simulink model "TV_2017"  (R2016a)
settings: Solver=FixedStepAuto  StartTime=0.0  StopTime=inf  FixedStep=0.001  RelTol=1e-3
PreLoadFcn:
  | TV_2017_parameters
values from neighbouring files (symbols this model uses):
  battery_voltage = single(530)    [HIL_parameters.m]    (also in HIL_parameters_2018.m; TV_2017_parameters.m; TV_2017_parameters_VD.m)
  car_params = Simulink_Car_params    [HIL_parameters.m]    (also in HIL_parameters_2018.m; TV_2017_parameters.m; TV_2017_parameters_VD.m)
  i_Diff = 16    [HIL_parameters.m]    (also in HIL_parameters_2018.m; TV_2017_parameters.m)
  Kp = 1    [HIL_parameters.m]    (also in HIL_parameters_2018.m; TV_2017_parameters.m; TV_2017_parameters_VD.m)
  motor_data = struct    [HIL_parameters.m]    (also in HIL_parameters_2018.m; TV_2017_parameters.m)
  powerLimitControl = Simulink_el    [HIL_parameters.m]    (also in HIL_parameters_2018.m; TV_2017_parameters.m; TV_2017_parameters_VD.m)
  settings = Simulink_Settings    [HIL_parameters.m]    (also in HIL_parameters_2018.m; TV_2017_parameters.m; TV_2017_parameters_VD.m)
  SpdC_BCC = 0    [HIL_parameters.m]    (also in HIL_parameters_2018.m; TV_2017_parameters.m; TV_2017_parameters_VD.m)
  Speed_Neg_sat = -21    [HIL_parameters.m]    (also in HIL_parameters_2018.m; TV_2017_parameters.m; TV_2017_parameters_VD.m)
  Speed_Pos_sat = 21    [HIL_parameters.m]    (also in HIL_parameters_2018.m; TV_2017_parameters.m; TV_2017_parameters_VD.m)
  SteeringAngleFL = [-23.80 -22.65 -21.50 -20.34 -19.18 -18.03 -16.86 -15.70 -14.53 -13.35 -12.18 -10.99 -9.80 -8.61 -7.40 -6.19 -4.97 -3.75 -2.51 -1.26 0 1.27 2.56 3.85 5.17 6.50 7.84 9.21 10.59 12.00 13.42 14.88 16.36 17.87 19.41 20.99 22.61 24.26 25.97 27.73 29.54]    [CarSetupAnalysis2018.m]    (also in HIL_parameters_2018.m; TV_2017_parameters.m; TV_2017_parameters_VD.m = [-24.129 -22.950 -21.772 -20.593 -19.413 -18.232 -17.050 -15)
  SteeringAngleFR = [-29.54 -27.73 -25.97 -24.26 -22.61 -20.99 -19.41 -17.87 -16.36 -14.88 -13.42 -12.00 -10.59 -9.21 -7.84 -6.50 -5.17 -3.85 -2.56 -1.27 0 1.26 2.51 3.75 4.97 6.19 7.40 8.61 9.80 10.99 12.18 13.35 14.53 15.70 16.86 18.03 19.18 20.34 21.50 22.65 23.80]    [CarSetupAnalysis2018.m]    (also in HIL_parameters_2018.m; TV_2017_parameters.m; TV_2017_parameters_VD.m = [-29.3050 -27.5340 -25.8140 -24.1410 -22.5110 -20.9180 -19.3)
  SteeringWhAngle = [-105 -99.75 -94.5 -89.25 -84 -78.75 -73.5 -68.25 -63 -57.75 -52.5 -47.25 -42 -36.75 -31.5 -26.25 -21.0 -15.75 -10.5 -5.25 0.0 5.25 10.50 15.75 21.00 26.25 31.50 36.75 42.00 47.25 52.50 57.75  63.00 68.25 73.50 78.75 84.00 89.25 94.50 99.75 105.00]    [TV_2017_parameters_VD.m]
  Tn_n = 0    [HIL_parameters.m]    (also in HIL_parameters_2018.m; TV_2017_parameters.m; TV_2017_parameters_VD.m)
  tractionControl = Simulink_tc    [HIL_parameters.m]    (also in HIL_parameters_2018.m; IterativeTractionControlTuning.m; TV_2017_parameters.m; TV_2017_parameters_VD.m)
  yawMomentGenerator = struct    [HIL_parameters.m]    (also in HIL_parameters_2018.m = Simulink_yawRate2; TV_2017_parameters.m = Simulink_yawRate2)
  yawRateControl = Simulink_yawRate    [HIL_parameters.m]    (also in HIL_parameters_2018.m; TV_2017_parameters.m; TV_2017_parameters_VD.m)
undefined symbols (not defined in the file or in its folder): DiscIntNeverNeededParam, magnitude, speedEstimation, TC_Decr_Gas, TC_Derivative, TC_Incr_Gas, TC_On, TC_Relay_Off, TC_Relay_On
libraries: CarMaker4SL x350, simulink_extras x63, simulink x37, dspfdesign x2
(part 3 of 14)

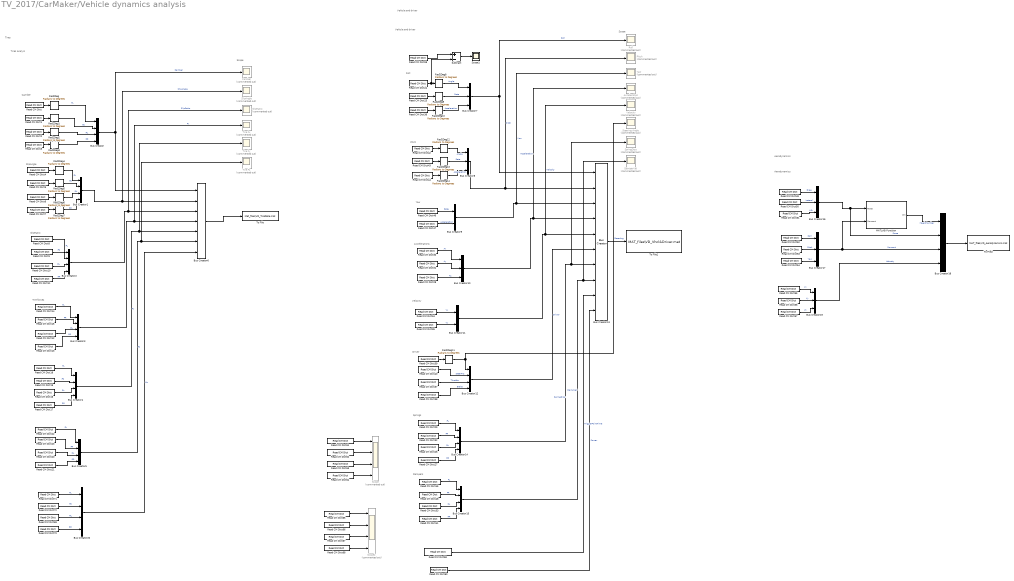
== system TV_2017/CarMaker/Vehicle dynamics analysis ==
  note: Aerodynamics
  note: Scope
  note: Scope
  note: Dampers
  note: Springs
  note: Driver
  note: Velocity
  note: Tire forces
  note: SlipRatio
  note: SlipAngle
  note: Camber
  note: Tires analyis
  note: Tires
  note: Accelerations
  note: Yaw
  note: Pitch
  note: Roll
  note: Vehicle and driver
  note: Vehicle and driver
  note: Aerodynamics
  Acceleration : Scope  Commented=on
  Bus Creator{,1..5,12,14..15,18,20} (11 alike) : BusCreator  Inputs=4
  Bus Creator{7..8,10,16..17,19} (6 alike) : BusCreator  Inputs=3
  Bus Creator11 : BusCreator  Inputs=2
  Bus Creator13 : BusCreator  Inputs=10
  Bus Creator6 : BusCreator  Inputs=7
  Bus Creator9 : BusCreator  Inputs=2
  Camber : Scope  Commented=on
  DamperVel : Scope  Commented=on
  MATLAB Function : MATLAB Function  TreatAsAtomicUnit=on
  Pitch : Scope  Commented=on
  Rad2Deg{,1..14} (15 alike) : simulink_extras/Transformations/Radians to Degrees
  Read CM Dict : CarMaker4SL/Read CM Dict  xname=Car.CamberFL  xsync=off
  Read CM Dict1 : CarMaker4SL/Read CM Dict  xname=Car.CamberFR  xsync=off
  Read CM Dict10 : CarMaker4SL/Read CM Dict  xname=Vhcl.RL.LongSlip  xsync=off
  Read CM Dict11 : CarMaker4SL/Read CM Dict  xname=Vhcl.RR.LongSlip  xsync=off
  Read CM Dict12 : CarMaker4SL/Read CM Dict  xname=Vhcl.RL.Fx  xsync=off
  Read CM Dict13 : CarMaker4SL/Read CM Dict  xname=Vhcl.RR.Fx  xsync=off
  Read CM Dict14 : CarMaker4SL/Read CM Dict  xname=Vhcl.FL.Fx  xsync=off
  Read CM Dict15 : CarMaker4SL/Read CM Dict  xname=Vhcl.FR.Fx  xsync=off
  Read CM Dict16 : CarMaker4SL/Read CM Dict  xname=Vhcl.RL.Fy  xsync=off
  Read CM Dict17 : CarMaker4SL/Read CM Dict  xname=Vhcl.RR.Fy  xsync=off
  Read CM Dict18 : CarMaker4SL/Read CM Dict  xname=Vhcl.FL.Fy  xsync=off
  Read CM Dict19 : CarMaker4SL/Read CM Dict  xname=Vhcl.FR.Fy  xsync=off
  Read CM Dict2 : CarMaker4SL/Read CM Dict  xname=Car.CamberRL  xsync=off
  Read CM Dict20 : CarMaker4SL/Read CM Dict  xname=Vhcl.RL.Fz  xsync=off
  Read CM Dict21 : CarMaker4SL/Read CM Dict  xname=Vhcl.RR.Fz  xsync=off
  Read CM Dict22 : CarMaker4SL/Read CM Dict  xname=Vhcl.FL.Fz  xsync=off
  Read CM Dict23 : CarMaker4SL/Read CM Dict  xname=Vhcl.FR.Fz  xsync=off
  Read CM Dict24 : CarMaker4SL/Read CM Dict  xname=Vhcl.Roll  xsync=off
  Read CM Dict25 : CarMaker4SL/Read CM Dict  xname=Vhcl.RollVel  xsync=off
  Read CM Dict26 : CarMaker4SL/Read CM Dict  xname=Car.SpringRL.l  xsync=off
  Read CM Dict27 : CarMaker4SL/Read CM Dict  xname=Car.SpringRR.l  xsync=off
  Read CM Dict28 : CarMaker4SL/Read CM Dict  xname=Car.az  xsync=off
  Read CM Dict29 : CarMaker4SL/Read CM Dict  xname=Car.SpringFL.l  xsync=off
  Read CM Dict3 : CarMaker4SL/Read CM Dict  xname=Car.CamberRR  xsync=off
  Read CM Dict30 : CarMaker4SL/Read CM Dict  xname=Car.ax  xsync=off
  Read CM Dict31 : CarMaker4SL/Read CM Dict  xname=Car.ay  xsync=off
  Read CM Dict32 : CarMaker4SL/Read CM Dict  xname=Car.SpringFR.l  xsync=off
  Read CM Dict33 : CarMaker4SL/Read CM Dict  xname=Car.DampRL.v  xsync=off
  Read CM Dict34 : CarMaker4SL/Read CM Dict  xname=Car.vx  xsync=off
  Read CM Dict35 : CarMaker4SL/Read CM Dict  xname=Car.vy  xsync=off
  Read CM Dict36 : CarMaker4SL/Read CM Dict  xname=Vhcl.RollAcc  xsync=off
  Read CM Dict37 : CarMaker4SL/Read CM Dict  xname=Driver.Gas  xsync=off
  Read CM Dict38 : CarMaker4SL/Read CM Dict  xname=Driver.Brake  xsync=off
  Read CM Dict39 : CarMaker4SL/Read CM Dict  xname=Vhcl.Steer.Ang  xsync=off
  Read CM Dict4 : CarMaker4SL/Read CM Dict  xname=Vhcl.FL.SideSlip  xsync=off
  Read CM Dict40 : CarMaker4SL/Read CM Dict  xname=Vhcl.Steer.Trq  xsync=off
  Read CM Dict41 : CarMaker4SL/Read CM Dict  xname=Car.DampRR.v  xsync=off
  Read CM Dict42 : CarMaker4SL/Read CM Dict  xname=Vhcl.Pitch  xsync=off
  Read CM Dict43 : CarMaker4SL/Read CM Dict  xname=Vhcl.PitchVel  xsync=off
  Read CM Dict44 : CarMaker4SL/Read CM Dict  xname=Vhcl.PitchAcc  xsync=off
  Read CM Dict45 : CarMaker4SL/Read CM Dict  xname=Car.DampFL.v  xsync=off
  Read CM Dict46 : CarMaker4SL/Read CM Dict  xname=Vhcl.YawRate  xsync=off
  Read CM Dict47 : CarMaker4SL/Read CM Dict  xname=Vhcl.YawAcc  xsync=off
  Read CM Dict48 : CarMaker4SL/Read CM Dict  xname=Car.DampFR.v  xsync=off
  Read CM Dict49 : CarMaker4SL/Read CM Dict  xname=Car.Aero.Frc_1.x  xsync=off
  Read CM Dict5 : CarMaker4SL/Read CM Dict  xname=Vhcl.FR.SideSlip  xsync=off
  Read CM Dict50 : CarMaker4SL/Read CM Dict  xname=Car.Aero.Frc_1.y  xsync=off
  Read CM Dict51 : CarMaker4SL/Read CM Dict  xname=Car.Aero.Frc_1.z  xsync=off
  Read CM Dict52 : CarMaker4SL/Read CM Dict  xname=Car.Aero.Trq_1.x  xsync=off
  Read CM Dict53 : CarMaker4SL/Read CM Dict  xname=Car.Aero.Trq_1.y  xsync=off
  Read CM Dict54 : CarMaker4SL/Read CM Dict  xname=Car.Aero.Trq_1.z  xsync=off
  Read CM Dict55 : CarMaker4SL/Read CM Dict  xname=Car.Aero.vres_1.x  xsync=off
  Read CM Dict56 : CarMaker4SL/Read CM Dict  xname=Car.Aero.vres_1.y  xsync=off
  Read CM Dict57 : CarMaker4SL/Read CM Dict  xname=Car.Aero.vres_1.z  xsync=off
  Read CM Dict58 : CarMaker4SL/Read CM Dict  xname=DM.TriggerPoint.Time  xsync=off
  Read CM Dict59 : CarMaker4SL/Read CM Dict  xname=Car.Roll  xsync=off
  Read CM Dict6 : CarMaker4SL/Read CM Dict  xname=Vhcl.RL.SideSlip  xsync=off
  Read CM Dict60 : CarMaker4SL/Read CM Dict  xname=Power  xsync=off
  Read CM Dict61 : CarMaker4SL/Read CM Dict  xname=Car.SpringFL.Frc_tot  xsync=off
  Read CM Dict62 : CarMaker4SL/Read CM Dict  xname=Car.SpringFR.Frc_tot  xsync=off
  Read CM Dict63 : CarMaker4SL/Read CM Dict  xname=Car.SpringRL.Frc_tot  xsync=off
  Read CM Dict64 : CarMaker4SL/Read CM Dict  xname=Car.SpringRR.Frc_tot  xsync=off
  Read CM Dict65 : CarMaker4SL/Read CM Dict  xname=Car.DampFL.Frc_tot  xsync=off
  Read CM Dict66 : CarMaker4SL/Read CM Dict  xname=Car.DampFR.Frc_tot  xsync=off
  Read CM Dict67 : CarMaker4SL/Read CM Dict  xname=Car.DampRL.Frc_tot  xsync=off
  Read CM Dict68 : CarMaker4SL/Read CM Dict  xname=Car.DampRR.Frc_tot  xsync=off
  Read CM Dict69 : CarMaker4SL/Read CM Dict  xname=Car.TrqAlignRL  xsync=off
  Read CM Dict7 : CarMaker4SL/Read CM Dict  xname=Vhcl.RR.SideSlip  xsync=off
  Read CM Dict70 : CarMaker4SL/Read CM Dict  xname=Car.TrqAlignRR  xsync=off
  Read CM Dict71 : CarMaker4SL/Read CM Dict  xname=Car.TrqAlignFL  xsync=off
  Read CM Dict72 : CarMaker4SL/Read CM Dict  xname=Car.TrqAlignFR  xsync=off
  Read CM Dict8 : CarMaker4SL/Read CM Dict  xname=Vhcl.FL.LongSlip  xsync=off
  Read CM Dict9 : CarMaker4SL/Read CM Dict  xname=Vhcl.FR.LongSlip  xsync=off
  Roll : Scope  Commented=on
  Scope : Scope  Commented=on  NumInputPorts=4
  Scope1 : Scope
  Scope2 : Scope  Commented=on  NumInputPorts=4
  SlipAngle : Scope  Commented=on
  SlipRatio : Scope  Commented=on
  SpringDisp : Scope  Commented=on
  Steering Angle : Scope  Commented=on
  Subtract : Sum  Inputs=+-
  Tire Fx : Scope  Commented=on
  Tire Fy : Scope  Commented=on
  Tire Fz : Scope  Commented=on
  To File : ToFile  Filename=Mat_files\VD_TireData.mat  MatrixName=Tire  SaveFormat=Timeseries
      settings: Decimation=2
  To File1 : ToFile  Filename=MAT_files\VD_Vhcl&Driver.mat  MatrixName=Vhcl  SaveFormat=Timeseries
      settings: Decimation=2
  To File2 : ToFile  Filename=MAT_files\VD_Aerodynamics.mat  MatrixName=Aero  SaveFormat=Timeseries
      settings: Decimation=2
  Velocity : Scope  Commented=on
  Yaw : Scope  Commented=on
  wires:
  Rad2Deg3/1 -> Bus Creator/4  "RR"
  Read CM Dict2/1 -> Rad2Deg2/1
  Rad2Deg/1 -> Bus Creator/1  "FL"
  Rad2Deg2/1 -> Bus Creator/3  "RL"
  Read CM Dict/1 -> Rad2Deg/1
  Rad2Deg1/1 -> Bus Creator/2  "FR"
  Read CM Dict1/1 -> Rad2Deg1/1
  Read CM Dict3/1 -> Rad2Deg3/1
  Rad2Deg7/1 -> Bus Creator1/4  "RR"
  Read CM Dict6/1 -> Rad2Deg6/1
  Rad2Deg4/1 -> Bus Creator1/1  "FL"
  Rad2Deg6/1 -> Bus Creator1/3  "RL"
  Read CM Dict4/1 -> Rad2Deg4/1
  Rad2Deg5/1 -> Bus Creator1/2  "FR"
  Read CM Dict5/1 -> Rad2Deg5/1
  Read CM Dict7/1 -> Rad2Deg7/1
  Read CM Dict11/1 -> Bus Creator2/4  "RR"
  Read CM Dict8/1 -> Bus Creator2/1  "FL"
  Read CM Dict10/1 -> Bus Creator2/3  "RL"
  Read CM Dict9/1 -> Bus Creator2/2  "FR"
  Read CM Dict13/1 -> Bus Creator3/4  "RR"
  Read CM Dict14/1 -> Bus Creator3/1  "FL"
  Read CM Dict12/1 -> Bus Creator3/3  "RL"
  Read CM Dict15/1 -> Bus Creator3/2  "FR"
  Read CM Dict17/1 -> Bus Creator4/4  "RR"
  Read CM Dict18/1 -> Bus Creator4/1  "FL"
  Read CM Dict16/1 -> Bus Creator4/3  "RL"
  Read CM Dict19/1 -> Bus Creator4/2  "FR"
  Read CM Dict21/1 -> Bus Creator5/4  "RR"
  Read CM Dict22/1 -> Bus Creator5/1  "FL"
  Read CM Dict20/1 -> Bus Creator5/3  "RL"
  Bus Creator/1 -> Bus Creator6/1, Camber/1  "Camber"
  Bus Creator1/1 -> SlipAngle/1, Bus Creator6/2  "SlipAngle"
  Bus Creator2/1 -> SlipRatio/1, Bus Creator6/3  "SlipRatio"
  Bus Creator3/1 -> Bus Creator6/4, Tire Fx/1  "Fx"
  Bus Creator4/1 -> Tire Fy/1, Bus Creator6/5  "Fy"
  Bus Creator5/1 -> Tire Fz/1, Bus Creator6/6  "Fz"
  Read CM Dict23/1 -> Bus Creator5/2  "FR"
  Bus Creator6/1 -> To File/1
  Read CM Dict36/1 -> Rad2Deg10/1
  Rad2Deg8/1 -> Bus Creator7/1  "Angle"
  Rad2Deg10/1 -> Bus Creator7/3  "Acceleration"
  Read CM Dict24/1 -> Subtract/2, Rad2Deg8/1
  Rad2Deg9/1 -> Bus Creator7/2  "Rate"
  Read CM Dict25/1 -> Rad2Deg9/1
  Read CM Dict44/1 -> Rad2Deg14/1
  Rad2Deg12/1 -> Bus Creator8/1  "Angle"
  Rad2Deg14/1 -> Bus Creator8/3  "Acceleration"
  Read CM Dict42/1 -> Rad2Deg12/1
  Rad2Deg13/1 -> Bus Creator8/2  "Rate"
  Read CM Dict43/1 -> Rad2Deg13/1
  Read CM Dict46/1 -> Bus Creator9/1  "Rate"
  Read CM Dict47/1 -> Bus Creator9/2  "Acceleration"
  Read CM Dict34/1 -> Bus Creator11/1  "Vx"
  Read CM Dict35/1 -> Bus Creator11/2  "Vy"
  Read CM Dict38/1 -> Bus Creator12/4  "Brake"
  Read CM Dict39/1 -> Rad2Deg11/1
  Read CM Dict37/1 -> Bus Creator12/3  "Throttle"
  Bus Creator7/1 -> Bus Creator13/1, Roll/1  "Roll"
  Bus Creator8/1 -> Pitch/1, Bus Creator13/2  "Pitch"
  Bus Creator9/1 -> Bus Creator13/3, Yaw/1  "Yaw"
  Bus Creator11/1 -> Velocity/1, Bus Creator13/5  "Velocity"
  Bus Creator12/1 -> Bus Creator13/6  "Driver"
  Read CM Dict40/1 -> Bus Creator12/2  "SteerTrq"
  Bus Creator13/1 -> To File1/1
  Rad2Deg11/1 -> Bus Creator12/1, Steering Angle/1  "SteerAng"
  Bus Creator10/1 -> Acceleration/1, Bus Creator13/4  "Acceleration"
  Read CM Dict27/1 -> Bus Creator14/4  "RR"
  Read CM Dict29/1 -> Bus Creator14/1  "FL"
  Read CM Dict26/1 -> Bus Creator14/3  "RL"
  Read CM Dict32/1 -> Bus Creator14/2  "FR"
  Bus Creator14/1 -> SpringDisp/1, Bus Creator13/7  "SpringDisp"
  Read CM Dict41/1 -> Bus Creator15/4  "RR"
  Read CM Dict45/1 -> Bus Creator15/1  "FL"
  Read CM Dict33/1 -> Bus Creator15/3  "RL"
  Read CM Dict48/1 -> Bus Creator15/2  "FR"
  Bus Creator15/1 -> DamperVel/1, Bus Creator13/8  "DampVel"
  Read CM Dict30/1 -> Bus Creator10/1  "Ax"
  Read CM Dict31/1 -> Bus Creator10/2  "Ay"
  Read CM Dict28/1 -> Bus Creator10/3  "Az"
  Read CM Dict49/1 -> Bus Creator16/1  "Drag"
  Read CM Dict50/1 -> Bus Creator16/2  "Lateral"
  Read CM Dict51/1 -> Bus Creator16/3  "Lift"
  Read CM Dict52/1 -> Bus Creator17/1  "Roll"
  Read CM Dict53/1 -> Bus Creator17/2  "Pitch"
  Read CM Dict54/1 -> Bus Creator17/3  "Yaw"
  Bus Creator16/1 -> Bus Creator18/2, MATLAB Function/1(Force)  "Force"
  Bus Creator17/1 -> MATLAB Function/2(Moment), Bus Creator18/3  "Moment"
  MATLAB Function/1(MM) -> Bus Creator18/1  "MagicMumber"
  Read CM Dict55/1 -> Bus Creator19/1  "Vx"
  Read CM Dict56/1 -> Bus Creator19/2  "Vy"
  Read CM Dict57/1 -> Bus Creator19/3  "Vz"
  Bus Creator19/1 -> Bus Creator18/4  "Velocity"
  Bus Creator18/1 -> To File2/1
  Read CM Dict59/1 -> Subtract/1
  Subtract/1 -> Scope1/1
  Read CM Dict60/1 -> Bus Creator13/10  "Power"
  Read CM Dict58/1 -> Bus Creator13/9  "TriggerPointTime"
  Read CM Dict61/1 -> Scope/1
  Read CM Dict62/1 -> Scope/2
  Read CM Dict63/1 -> Scope/3
  Read CM Dict64/1 -> Scope/4
  Read CM Dict65/1 -> Scope2/1
  Read CM Dict66/1 -> Scope2/2
  Read CM Dict67/1 -> Scope2/3
  Read CM Dict68/1 -> Scope2/4
  Read CM Dict70/1 -> Bus Creator20/4  "RR"
  Read CM Dict71/1 -> Bus Creator20/1  "FL"
  Read CM Dict69/1 -> Bus Creator20/3  "RL"
  Read CM Dict72/1 -> Bus Creator20/2  "FR"
  Bus Creator20/1 -> Bus Creator6/7  "Mz"

== system TV_2017/CarMaker/VehicleControl3 ==
  note: <Your model here>
  note: When implementing a vehicle control model,
      | be sure to add '-disablevehiclecontrol' to the command line arguments
      | in the CarMaker Model Configuration block.
      | Otherwise your model will possibly not see the original DrivMan signals
      | on its inputs, but those of a currently activated C-coded vehicle control model instead.
  Sync_In : Inport
  DrivMan.In : Inport  Port=2
  Bus Creator2 : BusCreator  Inputs=2
  CreateBus Vhcl.Misc : Subsystem
  CreateBus Vhcl.Wheel.In : Subsystem
  CreateBus VhclCtrl : Subsystem
  CreateBus VhclCtrl.PT : Subsystem
  CreateBus VhclCtrl.Steering : Subsystem
  Demux2 : Demux  Outputs=2
  VehicleControl : S-Function  FunctionName=CM_Sfun  Parameters='VehicleControl'  SFunctionDeploymentMode=off  EnableBusSupport=off
  VehicleControlUpd : S-Function  FunctionName=CM_Sfun  Parameters='VehicleControlUpd'  SFunctionDeploymentMode=off  EnableBusSupport=off
  Sync_Out : Outport
  Vhcl.Model.Source : Outport  Port=2
  VhclCtrl.Steering : Outport  Port=3
  Vhcl.Wheel.In : Outport  Port=4
  Vhcl.Misc : Outport  Port=5
  VhclCtrl.Brake : Outport  Port=6
  VhclCtrl.PT : Outport  Port=7
  wires:
  CreateBus VhclCtrl/1(Out) -> VehicleControlUpd/2
  VehicleControl/2 -> CreateBus VhclCtrl/1(In)
  VehicleControlUpd/2 -> Vhcl.Model.Source/1
  VehicleControlUpd/4 -> CreateBus Vhcl.Wheel.In/1(In1)
  VehicleControlUpd/5 -> CreateBus Vhcl.Misc/1(In1)
  VehicleControlUpd/6 -> Demux2/1
  VehicleControlUpd/7 -> CreateBus VhclCtrl.PT/1(In1)
  VehicleControlUpd/3 -> CreateBus VhclCtrl.Steering/1(In1)
  CreateBus Vhcl.Misc/1(Out1) -> Vhcl.Misc/1
  CreateBus Vhcl.Wheel.In/1(Out1) -> Vhcl.Wheel.In/1
  DrivMan.In/1 -> VehicleControl/2
  VehicleControl/1 -> VehicleControlUpd/1
  Sync_In/1 -> VehicleControl/1
  CreateBus VhclCtrl.PT/1(Out1) -> VhclCtrl.PT/1
  Bus Creator2/1 -> VhclCtrl.Brake/1
  CreateBus VhclCtrl.Steering/1(Out1) -> VhclCtrl.Steering/1
  VehicleControlUpd/1 -> Sync_Out/1
  Demux2/2 -> Bus Creator2/2  "VhclCtrl BrakePark"
  Demux2/1 -> Bus Creator2/1  "VhclCtrl Brake"

== system TV_2017/CarMaker/Control_System /Output Interface reduce slipratio ==
  Ti_lim : Inport
  MATLAB Function : MATLAB Function  TreatAsAtomicUnit=on
  "Ti_pos " : Outport
  Ti_neg : Outport  Port=2
  wi_setpoints : Outport  Port=3
  wires:
  MATLAB Function/2(Ti_neg) -> Ti_neg/1
  Ti_lim/1 -> MATLAB Function/1(Ti)
  MATLAB Function/1(Ti_pos) -> "Ti_pos "/1
  MATLAB Function/3(wi_setpoints) -> wi_setpoints/1

== system TV_2017/CarMaker/Control_System /Power Limit Torque Reduction Controller 2018 ==
  note: Hvis enable == 2, input 1 blir passet
      | Hvis Enable == {1,2}, input 3 blir passet
  Ti_lim : Inport
  states : Inport  Port=2
  Bus Creator1 : BusCreator  Inputs=4  OutDataTypeStr=Bus: Ti_lim  NonVirtualBus=on
      settings: InheritFromInputs=off
  Bus Creator2 : BusCreator  Inputs=4  OutDataTypeStr=Bus: Motor_Efficiencies  NonVirtualBus=on
      settings: InheritFromInputs=off
  Delay : Delay  DelayLength=1
  Motorestimates : Subsystem
  "Old powerlimiting " : Subsystem  Commented=on
  Powerlimiting_Control_block : MATLAB Function  TreatAsAtomicUnit=on  SystemSampleTime=0.01
  Scope1 : Scope  NumInputPorts=2
  Scope2 : Scope  NumInputPorts=4
  Scope3 : Scope  NumInputPorts=4
  Scope4 : Scope
  Scope8 : Scope  NumInputPorts=5
  To Workspace : ToWorkspace  VariableName=Powertest  SaveFormat=Timeseries  SampleTime=-1
  extractPower1 : MATLAB Function  TreatAsAtomicUnit=on
  t_lim : Outport
  Efficiency : Outport  Port=2
  wires:
  states/1 -> Powerlimiting_Control_block/1(states), extractPower1/1(states), "Old powerlimiting "/2(states), Motorestimates/1(states)
  Powerlimiting_Control_block/3(RL) -> Bus Creator1/3, Scope8/3
  Powerlimiting_Control_block/1(FL) -> Scope8/1, Bus Creator1/1
  Powerlimiting_Control_block/4(RR) -> Scope8/4, Bus Creator1/4
  Ti_lim/1 -> "Old powerlimiting "/1(ti_lim), Delay/1, t_lim/1, Powerlimiting_Control_block/3(Ti_lim)
  Motorestimates/1(Eff_FL) -> Scope2/1, Bus Creator2/1
  Motorestimates/2(Eff_FR) -> Bus Creator2/2
  Motorestimates/3(Eff_RL) -> Bus Creator2/3
  Motorestimates/4(Eff_RR) -> Bus Creator2/4
  Bus Creator2/1 -> Efficiency/1, Powerlimiting_Control_block/2(Motor_Efficiencies)
  extractPower1/1(power) -> To Workspace/1, Scope1/2
  Powerlimiting_Control_block/6(test1) -> Scope3/1
  Powerlimiting_Control_block/5(state) -> Scope4/1
  Powerlimiting_Control_block/2(FR) -> Bus Creator1/2, Scope8/2
  Delay/1 -> Motorestimates/2(Ti_lim)

== system TV_2017/CarMaker/Control_System /Slip Rate Control  ==
  Ti_ref : Inport
  "States " : Inport  Port=2
  T_req : Inport  Port=3
  Bus Selector : BusSelector  OutputSignals=FL,FR,RL,RR
  Constant : Constant  Value=0
  Index Vector : MultiPortSwitch  DataPortOrder=Zero-based contiguous  Inputs=2  zeroidx=on
  Mux18 : Mux
  SMC Traction Control : Subsystem  Commented=on
  SUM : Subsystem
  Traction Controllers : Subsystem
  tcOutput : Scope
  Ti_lim : Outport
  T_sum_TC : Outport  Port=2
  wires:
  "States "/1 -> Traction Controllers/1(states)
  Ti_ref/1 -> Traction Controllers/2(Ti_ref), Index Vector/2
  Index Vector/1 -> Ti_lim/1
  Constant/1 -> Index Vector/1
  T_req/1 -> Traction Controllers/3(T_requested)
  Mux18/1 -> tcOutput/1
  Bus Selector/1 -> Mux18/1  "<FL>"
  Bus Selector/2 -> Mux18/2  "<FR>"
  Bus Selector/3 -> Mux18/3  "<RL>"
  Bus Selector/4 -> Mux18/4  "<RR>"
  Traction Controllers/1(Ti_SR) -> SUM/1(In1), Bus Selector/1, Index Vector/3
  SUM/1(Out1) -> T_sum_TC/1

== system TV_2017/CarMaker/Control_System /Subsystem ==
  In1 : Inport
  In2 : Inport  Port=2
  In3 : Inport  Port=3
  In4 : Inport  Port=4
  In5 : Inport  Port=5
  In6 : Inport  Port=6
  In7 : Inport  Port=7
  In8 : Inport  Port=8
  In9 : Inport  Port=9
  In10 : Inport  Port=10
  In11 : Inport  Port=11
  In12 : Inport  Port=12
  In13 : Inport  Port=13
  In14 : Inport  Port=14
  In15 : Inport  Port=15
  In16 : Inport  Port=16
  In17 : Inport  Port=17
  In18 : Inport  Port=18
  In19 : Inport  Port=19
  2016 adapted : Subsystem  Commented=on
  OutputTelemetri : MATLAB Function  Commented=on  TreatAsAtomicUnit=on
  Torque allocation 2016 : Subsystem  Commented=on
  Torque allocation 2017 : Subsystem  Commented=on
  Torque allocation QP- : Subsystem  Commented=on
  Torque allocation QP-1 : Subsystem  Commented=on
  Out1 : Outport
  Out2 : Outport  Port=2
  Out3 : Outport  Port=3
  Out4 : Outport  Port=4
  Out5 : Outport  Port=5
  Out6 : Outport  Port=6
  Out7 : Outport  Port=7
  Out8 : Outport  Port=8
  Out9 : Outport  Port=9
  Out10 : Outport  Port=10
  Out11 : Outport  Port=11
  Out12 : Outport  Port=12
  Out13 : Outport  Port=13
  Out14 : Outport  Port=14
  Out15 : Outport  Port=15
  Out16 : Outport  Port=16
  Out17 : Outport  Port=17
  Out18 : Outport  Port=18
  Out19 : Outport  Port=19
  Out20 : Outport  Port=20
  Out21 : Outport  Port=21
  Out22 : Outport  Port=22
  Out23 : Outport  Port=23
  Out24 : Outport  Port=24
  wires:
  2016 adapted/3(saturated_constraints) -> Out12/1
  In4/1 -> Torque allocation QP-/2(T_req)
  Torque allocation QP-/1("Mz_allocated ") -> Out1/1
  Torque allocation QP-/4(max_motor_torque) -> Out6/1
  In17/1 -> Torque allocation QP-1/2(T_req)
  In19/1 -> Torque allocation QP-1/3("States ")
  Torque allocation QP-1/2(Ti_lim) -> Out18/1
  Torque allocation QP-1/4(max_motor_torque) -> Out21/1
  2016 adapted/2(Ti_lim) -> Out10/1
  2016 adapted/1("Mz_allocated ") -> Out9/1
  In1/1 -> Torque allocation 2016/1(Mz_ref)
  In3/1 -> Torque allocation 2016/2(T_req)
  Torque allocation QP-/5(active_constraints) -> Out8/1
  In5/1 -> Torque allocation 2016/3("States ")
  Torque allocation QP-1/3(saturated_constraints) -> Out20/1
  2016 adapted/4(Max_motor_torque) -> Out13/1
  In6/1 -> Torque allocation QP-/3("States ")
  Torque allocation QP-1/5(active_constraints) -> Out23/1
  Torque allocation 2016/1(Ti_lim) -> Out2/1
  Torque allocation QP-/2(Ti_lim) -> Out3/1
  Torque allocation QP-/3(saturated_constraints) -> Out5/1
  In15/1 -> Torque allocation QP-1/1(Mz_ref)
  Torque allocation QP-1/1("Mz_allocated ") -> Out16/1
  In12/1 -> 2016 adapted/3("States ")
  In8/1 -> 2016 adapted/1(Mz_ref)
  In2/1 -> Torque allocation QP-/1(Mz_ref)
  2016 adapted/5(active_constraints) -> Out14/1
  In10/1 -> 2016 adapted/2(T_req)
  Torque allocation 2017/1("Mz_allocated ") -> Out15/1
  In9/1 -> OutputTelemetri/2(T_req)
  In18/1 -> Torque allocation 2017/3("States ")
  Torque allocation 2017/5(active_constraints) -> Out24/1
  In7/1 -> OutputTelemetri/1(states)
  In11/1 -> OutputTelemetri/3(r_ref)
  Torque allocation 2017/3(saturated_constraints) -> Out19/1
  Torque allocation 2017/2(Ti_lim) -> Out17/1
  In16/1 -> Torque allocation 2017/2(T_req)
  Torque allocation 2016/2("Mz_error ") -> Out4/1
  In14/1 -> Torque allocation 2017/1(Mz_ref)
  Torque allocation 2017/4(max_motor_torque) -> Out22/1
  Torque allocation 2016/3(Max_motor_torque_i) -> Out7/1
  In13/1 -> OutputTelemetri/4(Mz_ref_to_telemetry)
  OutputTelemetri/1(OutputTelemetri_control) -> Out11/1

== system TV_2017/CarMaker/Control_System /TA 2017 ==
  Mz_ref : Inport
  T_req : Inport  Port=2
  "States " : Inport  Port=3
  "Motoreff " : Inport  Port=4
  Bus Selector : BusSelector  OutputSignals=Efficiency_FL,Efficiency_FR,Efficiency_RL,Efficiency_RR
  Bus Selector1 : BusSelector  OutputSignals=mmt_FL,mmt_FR,mmt_RL,mmt_RR
  Bus Selector2 : BusSelector  OutputSignals=mmt_FL,mmt_FR,mmt_RL,mmt_RR
  Bus Selector3 : BusSelector  OutputSignals=FL,FR,RL,RR
  Bus Selector6 : BusSelector  OutputSignals=FL,FR,RL,RR
  Friction Torque Limits : Scope
  Mux{1..5,7} (6 alike) : Mux
  Mz : Scope
  Mz1 : Scope
  "Slip handling (Traction Control) " : Subsystem
  SlipScalingFactor : Scope
  Ti_Lim_TA : Scope
  Ti_Lim_TA1 : Scope
  Ti_max : Scope
  To Workspace : ToWorkspace  VariableName=efficiency  SampleTime=-1
      settings: Save2DSignal=2-D array (concatenate along first dimension)
  Torque lim Slip : Scope
  TorqueAllocation : MATLAB Function  TreatAsAtomicUnit=on
  TorqueLimFZ : Scope
  "max combined tire torque based on (Fz, SA,mu) " : MATLAB Function  TreatAsAtomicUnit=on
  "max long tire torque based on (FZ , mu)" : MATLAB Function  TreatAsAtomicUnit=on
  "max torque " : MATLAB Function  TreatAsAtomicUnit=on
  required torque : Scope  NumInputPorts=4
  "Mz_error " : Outport
  Ti_lim : Outport  Port=2
  pow_red : Outport  Port=3
  max_motor_torque : Outport  Port=4
  active_constraints : Outport  Port=5
  overiterate 1 : Outport  Port=6
  wires:
  Mux1/1 -> Mz/1
  TorqueAllocation/4(Mz_allocated) -> required torque/4, Mux1/2  "Mz_all"
  TorqueAllocation/2(pow_red) -> pow_red/1, Ti_max/1
  Mz_ref/1 -> required torque/2, Mux1/3, TorqueAllocation/1(Mz_ref)  "Mz_ref"
  "States "/1 -> [states], TorqueAllocation/3(states)
  "max torque "/2(active_constraints) -> [active_constraints]
  "max long tire torque based on (FZ , mu)"/1(maxMotorTorque) -> Bus Selector2/1, "max torque "/1(mu_lim)
  [maxMotorTorque] -> max_motor_torque/1
  [active_constraints] -> active_constraints/1
  "max torque "/1(maxMotorTorque) -> [maxMotorTorque]
  [maxMotorTorque] -> TorqueAllocation/4(maxMotorTorque)
  TorqueAllocation/3(Mz_error) -> required torque/3, "Mz_error "/1, Mux1/1  "Mz_error"
  "max torque "/3(friction_limits) -> Friction Torque Limits/1, [friction_torque_limits]
  [friction_torque_limits] -> TorqueAllocation/5(friction_limit_torques)
  TorqueAllocation/5(overiterate) -> overiterate 1/1
  "max combined tire torque based on (Fz, SA,mu) "/1(maxMotorTorque) -> "max torque "/4(mot_temp_lim), "max torque "/3(inv_temp_lim), "max torque "/2(SA_lim), Bus Selector1/1
  [states] -> "Slip handling (Traction Control) "/1(Sensors), "max long tire torque based on (FZ , mu)"/1(states), "max combined tire torque based on (Fz, SA,mu) "/1(states)
  Bus Selector6/1 -> Mux7/1  "<FL>"
  Bus Selector6/2 -> Mux7/2  "<FR>"
  Bus Selector6/3 -> Mux7/3  "<RL>"
  Bus Selector6/4 -> Mux7/4  "<RR>"
  TorqueAllocation/1(Ti_lim) -> Bus Selector6/1, Ti_lim/1
  Mux7/1 -> Ti_Lim_TA/1
  Bus Selector1/1 -> Mux2/1  "<mmt_FL>"
  Bus Selector1/2 -> Mux2/2  "<mmt_FR>"
  Bus Selector1/3 -> Mux2/3  "<mmt_RL>"
  Bus Selector1/4 -> Mux2/4  "<mmt_RR>"
  Mux2/1 -> Torque lim Slip/1
  Bus Selector2/1 -> Mux3/1  "<mmt_FL>"
  Bus Selector2/2 -> Mux3/2  "<mmt_FR>"
  Bus Selector2/3 -> Mux3/3  "<mmt_RL>"
  Bus Selector2/4 -> Mux3/4  "<mmt_RR>"
  Mux3/1 -> TorqueLimFZ/1
  Bus Selector3/1 -> Mux4/1  "<FL>"
  Bus Selector3/2 -> Mux4/2  "<FR>"
  Bus Selector3/3 -> Mux4/3  "<RL>"
  Bus Selector3/4 -> Mux4/4  "<RR>"
  Mux4/1 -> SlipScalingFactor/1
  "Slip handling (Traction Control) "/1(slipScalingFactors) -> "max torque "/5(slipScalingFactors), Bus Selector3/1
  T_req/1 -> required torque/1, Mux1/4, TorqueAllocation/2(T_req)
  "Motoreff "/1 -> Bus Selector/1, TorqueAllocation/6(Motoreff)
  Bus Selector/1 -> Mux5/1  "<Efficiency_FL>"
  Bus Selector/2 -> Mux5/2  "<Efficiency_FR>"
  Bus Selector/3 -> Mux5/3  "<Efficiency_RL>"
  Bus Selector/4 -> Mux5/4  "<Efficiency_RR>"
  Mux5/1 -> To Workspace/1, Ti_Lim_TA1/1

== system TV_2017/CarMaker/Control_System /Yaw_rate_Mz_generator ==
  Mz_error : Inport
  States : Inport  Port=2
  Enable/disable : Constant  Value=yawRateControl.method
  "Mz_1 , Mz_2" : Scope  NumInputPorts=2
  Switch : Switch  Threshold=1.5
  Switch1 : Switch  Criteria=u2 > Threshold
  "Yaw Rate Controller " : Subsystem
  Yaw Rate Generator : Subsystem
  Mz_Ref : Outport
  r_ref : Outport  Port=2
  wires:
  "Yaw Rate Controller "/3(Mz_ref) -> "Mz_1 , Mz_2"/1, Switch/1
  "Yaw Rate Controller "/1("r_ref ") -> r_ref/1  "r_ref"
  "Yaw Rate Controller "/4(Mz_ref_to_telemetry) -> Switch1/1
  Yaw Rate Generator/1(Mz_ref) -> "Mz_1 , Mz_2"/2, Switch/3
  Yaw Rate Generator/2(Mz_ref_to_telemetry) -> Switch1/3
  States/1 -> "Yaw Rate Controller "/2(States), Yaw Rate Generator/1(States)
  Mz_error/1 -> "Yaw Rate Controller "/1("Mz_error ")
  Switch/1 -> Mz_Ref/1
  Switch1/1 -> [Mz_ref_tt]
  Enable/disable/1 -> Switch1/2, Switch/2

== system TV_2017/CarMaker/Debug Information /Extract and scale to deg compare to CM output in individual error ==
  SA_CM : Inport
  In1 : Inport  Port=2
  Bus Selector1 : BusSelector  OutputSignals=FL,FR,RL,RR
  Demux : Demux
  Rate Transition2 : RateTransition  OutPortSampleTime=0.001
  SA  estimate : Scope  NumInputPorts=4
  Sum{,1..3} (4 alike) : Sum  Inputs=|-+
  r2d{,1..3} (4 alike) : simulink_extras/Transformations/Radians to Degrees
  FL : Outport
  FR : Outport  Port=2
  RL : Outport  Port=3
  RR : Outport  Port=4
  wires:
  SA_CM/1 -> Demux/1
  Demux/1 -> Sum/1
  r2d/1 -> Sum/2, SA  estimate/1
  Demux/2 -> Sum1/1
  r2d1/1 -> Sum1/2, SA  estimate/2
  Demux/3 -> Sum2/1
  r2d2/1 -> Sum2/2, SA  estimate/3
  Demux/4 -> Sum3/1
  r2d3/1 -> SA  estimate/4, Sum3/2
  Sum/1 -> FL/1
  Sum1/1 -> FR/1
  Sum2/1 -> RL/1
  Sum3/1 -> RR/1
  In1/1 -> Rate Transition2/1
  Bus Selector1/1 -> r2d/1  "<FL>"
  Bus Selector1/2 -> r2d1/1  "<FR>"
  Bus Selector1/3 -> r2d2/1  "<RL>"
  Bus Selector1/4 -> r2d3/1  "<RR>"
  Rate Transition2/1 -> Bus Selector1/1

== system TV_2017/CarMaker/Debug Information /Extract and scale to deg compare to CM output in individual error1 ==
  SA_CM : Inport
  In1 : Inport  Port=2
  Bus Selector1 : BusSelector  OutputSignals=SR_FL,SR_FR,SR_RL,SR_RR
  Demux : Demux
  Rate Transition2 : RateTransition  OutPortSampleTime=0.001
  SR  estimate : Scope  NumInputPorts=4
  Sum{,1..3} (4 alike) : Sum  Inputs=|-+
  r2d{,1..3} (4 alike) : simulink_extras/Transformations/Radians to Degrees  Commented=on
  FL : Outport
  FR : Outport  Port=2
  RL : Outport  Port=3
  RR : Outport  Port=4
  wires:
  SA_CM/1 -> Demux/1
  Demux/1 -> Sum/1
  Demux/2 -> Sum1/1
  Demux/3 -> Sum2/1
  Demux/4 -> Sum3/1
  Sum/1 -> FL/1
  Sum1/1 -> FR/1
  Sum2/1 -> RL/1
  Sum3/1 -> RR/1
  In1/1 -> Rate Transition2/1
  Bus Selector1/1 -> Sum/2, SR  estimate/1  "<SR_FL>"
  Bus Selector1/2 -> Sum1/2, SR  estimate/2  "<SR_FR>"
  Bus Selector1/3 -> Sum2/2, SR  estimate/3  "<SR_RL>"
  Bus Selector1/4 -> SR  estimate/4, Sum3/2  "<SR_RR>"
  Rate Transition2/1 -> Bus Selector1/1

== system TV_2017/CarMaker/Debug Information /Fz_Estimation ==
  sensors : Inport
  v_x : Inport  Port=2
  Bus Selector : BusSelector  OutputSignals=damper_rate_FL,damper_rate_FR,damper_rate_RL,damper_rate_RR
  Bus Selector1 : BusSelector  OutputSignals=FL,FR,RL,RR
  Bus Selector2 : BusSelector  OutputSignals=FL,FR,RL,RR
  Constant : Constant  Value=settings.select_Fz_est_method
  DamperRateLookup : Lookup_n-D  NumberOfTableDimensions=1  BreakpointsForDimension1=car_params.damper_table_breakpoint;  Table=car_params.damper_pull_push_values_front;  ExtrapMethod=Clip  UseLastTableValue=on  InternalRulePriority=Speed  RndMeth=Simplest  InputSameDT=on
  DamperRateLookup1 : Lookup_n-D  NumberOfTableDimensions=1  BreakpointsForDimension1=car_params.damper_table_breakpoint;  Table=car_params.damper_pull_push_values_front;  ExtrapMethod=Clip  UseLastTableValue=on  InternalRulePriority=Speed  RndMeth=Simplest  InputSameDT=on
  DamperRateLookup2 : Lookup_n-D  NumberOfTableDimensions=1  BreakpointsForDimension1=car_params.damper_table_breakpoint;  Table=car_params.damper_pull_push_values_rear;  ExtrapMethod=Clip  UseLastTableValue=on  InternalRulePriority=Speed  RndMeth=Simplest  InputSameDT=on
  DamperRateLookup3 : Lookup_n-D  NumberOfTableDimensions=1  BreakpointsForDimension1=car_params.damper_table_breakpoint;  Table=car_params.damper_pull_push_values_rear;  ExtrapMethod=Clip  UseLastTableValue=on  InternalRulePriority=Speed  RndMeth=Simplest  InputSameDT=on
  DamperRateLookup4 : Lookup_n-D  Commented=on  NumberOfTableDimensions=1  BreakpointsForDimension1=single([-200,0,200]);  Table=single([-500,0,500]);  ExtrapMethod=Clip  UseLastTableValue=on  InternalRulePriority=Speed  RndMeth=Simplest  InputSameDT=on
  DamperRateLookup5 : Lookup_n-D  Commented=on  NumberOfTableDimensions=1  BreakpointsForDimension1=single([-200,0,200]);  Table=single([-500,0,500]);  ExtrapMethod=Clip  UseLastTableValue=on  InternalRulePriority=Speed  RndMeth=Simplest  InputSameDT=on
  FzEstDamper : MATLAB Function  TreatAsAtomicUnit=on
  FzEstDamper 2016 : MATLAB Function  Commented=on  TreatAsAtomicUnit=on
  FzEstLoadTransfer : MATLAB Function  TreatAsAtomicUnit=on
  Index Vector : MultiPortSwitch  Inputs=2
  Scope : Scope  NumInputPorts=4
  Scope1 : Scope  NumInputPorts=4
  Fz_est : Outport
  Fz_LoadTransfer_est : Outport  Port=2
  Fz_damper_est : Outport  Port=3
  alfa_r : Outport  Port=4
  wires:
  sensors/1 -> FzEstLoadTransfer/1(sensor), FzEstDamper/1(sensors), Bus Selector/1
  DamperRateLookup/1 -> FzEstDamper/2(Fz_damp_FL)  "Fz_damp_FL"
  Bus Selector/1 -> DamperRateLookup/1  "<damper_rate_FL>"
  Bus Selector/2 -> DamperRateLookup1/1  "<damper_rate_FR>"
  Bus Selector/3 -> DamperRateLookup2/1  "<damper_rate_RL>"
  Bus Selector/4 -> DamperRateLookup3/1  "<damper_rate_RR>"
  DamperRateLookup1/1 -> FzEstDamper/3(Fz_damp_FR)
  DamperRateLookup2/1 -> FzEstDamper/4(Fz_damp_RL)
  DamperRateLookup3/1 -> FzEstDamper/5(Fz_damp_RR)
  Index Vector/1 -> Fz_est/1
  v_x/1 -> FzEstLoadTransfer/2(vx)
  FzEstDamper/2(alfa_r) -> alfa_r/1
  Bus Selector1/2 -> Scope/2  "<FR>"
  Bus Selector1/1 -> Scope/1  "<FL>"
  Bus Selector1/3 -> Scope/3  "<RL>"
  Bus Selector1/4 -> Scope/4  "<RR>"
  Constant/1 -> Index Vector/1
  FzEstLoadTransfer/1(Fz_loadTransfer_est) -> Bus Selector2/1, Fz_LoadTransfer_est/1, Index Vector/2
  Bus Selector2/2 -> Scope1/2  "<FR>"
  Bus Selector2/1 -> Scope1/1  "<FL>"
  Bus Selector2/3 -> Scope1/3  "<RL>"
  Bus Selector2/4 -> Scope1/4  "<RR>"
  FzEstDamper/1(Fz_damper_est) -> Index Vector/3, Bus Selector1/1, Fz_damper_est/1
  DamperRateLookup4/1 -> FzEstDamper 2016/3(Fz_damp_FR)
  DamperRateLookup5/1 -> FzEstDamper 2016/4(Fz_damp_RL)

== system TV_2017/CarMaker/Debug Information /Mechanical effect ==
  Gain{8,16..17,19} (4 alike) : Gain  Gain=1/car_params.GR
  Gain{18,20..22} (4 alike) : Gain  Gain=car_params.GR
  Mux7 : Mux
  Pmechanical : Scope
  Product{,1..3} (4 alike) : Product
  Read CM Dict12 : CarMaker4SL/Read CM Dict  xname=Car.WheelSpd_RL  xsync=off
  Read CM Dict13 : CarMaker4SL/Read CM Dict  xname=Car.WheelSpd_FR  xsync=off
  Read CM Dict14 : CarMaker4SL/Read CM Dict  xname=Car.WheelSpd_FL  xsync=off
  Read CM Dict15 : CarMaker4SL/Read CM Dict  xname=PT.WFL.Trq_Drive  xsync=off
  Read CM Dict16 : CarMaker4SL/Read CM Dict  xname=Car.WheelSpd_RR  xsync=off
  Read CM Dict45 : CarMaker4SL/Read CM Dict  xname=PT.WFR.Trq_Drive  xsync=off
  Read CM Dict46 : CarMaker4SL/Read CM Dict  xname=PT.WRL.Trq_Drive  xsync=off
  Read CM Dict47 : CarMaker4SL/Read CM Dict  xname=PT.WRR.Trq_Drive  xsync=off
  To File10 : ToFile  Filename=MAT_files\MechanicalEffect.mat  MatrixName=MechEffect  SaveFormat=Timeseries
  wires:
  Mux7/1 -> Pmechanical/1, To File10/1
  Read CM Dict12/1 -> Gain18/1
  Gain17/1 -> Product1/1
  Read CM Dict14/1 -> Gain22/1
  Gain16/1 -> Product2/1
  Read CM Dict16/1 -> Gain20/1
  Gain19/1 -> Product/1
  Read CM Dict15/1 -> Gain16/1
  Read CM Dict45/1 -> Gain17/1
  Gain8/1 -> Product3/1
  Product1/1 -> Mux7/2  "FR"
  Product/1 -> Mux7/3  "RL"
  Gain22/1 -> Product2/2
  Gain21/1 -> Product1/2
  Read CM Dict47/1 -> Gain8/1
  Product3/1 -> Mux7/4  "RR"
  Read CM Dict13/1 -> Gain21/1
  Gain18/1 -> Product/2
  Gain20/1 -> Product3/2
  Read CM Dict46/1 -> Gain19/1
  Product2/1 -> Mux7/1  "FL"

== system TV_2017/CarMaker/Debug Information /SA calculation ==
  In1 : Inport
  Bus Selector2 : BusSelector  OutputSignals=steering_wheel_angle
  Degrees to Radians : simulink_extras/Transformations/Degrees to Radians
  Degrees to Radians1 : simulink_extras/Transformations/Degrees to Radians
  FL steer ang lookup deg : Lookup_n-D  NumberOfTableDimensions=1  BreakpointsForDimension1=SteeringAngleFL  Table=SteeringAngleFL  ExtrapMethod=Clip  UseLastTableValue=on  InternalRulePriority=Speed  RndMeth=Simplest  InputSameDT=on
  FR steer ang lookup deg : Lookup_n-D  NumberOfTableDimensions=1  BreakpointsForDimension1=SteeringAngleFR  Table=SteeringAngleFR  ExtrapMethod=Clip  UseLastTableValue=on  InternalRulePriority=Speed  RndMeth=Simplest  InputSameDT=on
  Radians to Degrees1 : simulink_extras/Transformations/Radians to Degrees
  Slip angle calc : MATLAB Function  TreatAsAtomicUnit=on
  Out1 : Outport
  wires:
  Radians to Degrees1/1 -> FL steer ang lookup deg/1, FR steer ang lookup deg/1
  Degrees to Radians1/1 -> Slip angle calc/2(wheel_ang_right)
  Slip angle calc/1(SA) -> Out1/1
  FR steer ang lookup deg/1 -> Degrees to Radians1/1
  Degrees to Radians/1 -> Slip angle calc/1(wheel_ang_left)
  In1/1 -> Slip angle calc/3(sensor), Bus Selector2/1
  FL steer ang lookup deg/1 -> Degrees to Radians/1
  Bus Selector2/1 -> Radians to Degrees1/1  "<steering_wheel_angle>"

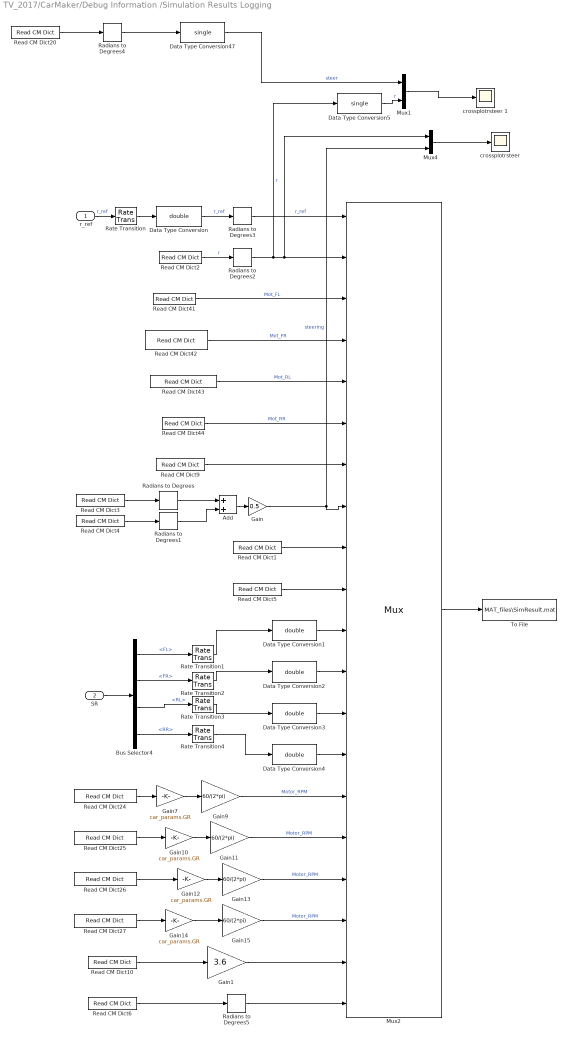
== system TV_2017/CarMaker/Debug Information /Simulation Results Logging ==
  r_ref : Inport
  SR : Inport  Port=2
  Add : Sum
  Bus Selector4 : BusSelector  OutputSignals=FL,FR,RL,RR
  Data Type Conversion{,1..4} (5 alike) : DataTypeConversion  OutDataTypeStr=double
  Data Type Conversion47 : DataTypeConversion  OutDataTypeStr=single
  Data Type Conversion5 : DataTypeConversion  OutDataTypeStr=single
  Gain : Gain  Gain=0.5
  Gain1 : Gain  Gain=3.6
  Gain{7,10,12,14} (4 alike) : Gain  Gain=car_params.GR
  Gain{9,11,13,15} (4 alike) : Gain  Gain=60/(2*pi)
  Mux1 : Mux  Inputs=2
  Mux2 : Mux  Inputs=20
  Mux4 : Mux  Inputs=2
  Radians to Degrees{,1..5} (6 alike) : simulink_extras/Transformations/Radians to Degrees
  Rate Transition{,1..4} (5 alike) : RateTransition  OutPortSampleTime=0.001
  Read CM Dict1 : CarMaker4SL/Read CM Dict  xname=Vhcl.Fr1.x  xsync=off
  Read CM Dict10 : CarMaker4SL/Read CM Dict  xname=Car.vx  xsync=off
  Read CM Dict2 : CarMaker4SL/Read CM Dict  xname=Car.YawRate  xsync=off
  Read CM Dict20 : CarMaker4SL/Read CM Dict  xname=Vhcl.Steer.Ang  xsync=off
  Read CM Dict24 : CarMaker4SL/Read CM Dict  xname=Car.WheelSpd_FL  xsync=off
  Read CM Dict25 : CarMaker4SL/Read CM Dict  xname=Car.WheelSpd_FR  xsync=off
  Read CM Dict26 : CarMaker4SL/Read CM Dict  xname=Car.WheelSpd_RL  xsync=off
  Read CM Dict27 : CarMaker4SL/Read CM Dict  xname=Car.WheelSpd_RR  xsync=off
  Read CM Dict3 : CarMaker4SL/Read CM Dict  xname=Car.CFR.rz  xsync=off
  Read CM Dict4 : CarMaker4SL/Read CM Dict  xname=Car.CFL.rz  xsync=off
  Read CM Dict41 : CarMaker4SL/Read CM Dict  xname=PT.WFL.Trq_Drive  xsync=off
  Read CM Dict42 : CarMaker4SL/Read CM Dict  xname=PT.WFR.Trq_Drive  xsync=off
  Read CM Dict43 : CarMaker4SL/Read CM Dict  xname=PT.WRL.Trq_Drive  xsync=off
  Read CM Dict44 : CarMaker4SL/Read CM Dict  xname=PT.WRR.Trq_Drive  xsync=off
  Read CM Dict5 : CarMaker4SL/Read CM Dict  xname=Vhcl.Fr1.y  xsync=off
  Read CM Dict6 : CarMaker4SL/Read CM Dict  xname=Vhcl.Steer.Ang  xsync=off
  Read CM Dict9 : CarMaker4SL/Read CM Dict  xname=Car.ay  xsync=off
  To File : ToFile  Filename=MAT_files\SimResult.mat  MatrixName=sim  SaveFormat=Timeseries
  "crossplotrsteer " : Scope
  crossplotrsteer 1 : Scope
  wires:
  r_ref/1 -> Rate Transition/1  "r_ref"
  Read CM Dict2/1 -> Radians to Degrees2/1  "r"
  Data Type Conversion/1 -> Radians to Degrees3/1  "r_ref"
  Read CM Dict42/1 -> Mux2/4  "Mot_FR"
  Read CM Dict43/1 -> Mux2/5  "Mot_RL"
  Read CM Dict41/1 -> Mux2/3  "Mot_FL"
  Read CM Dict44/1 -> Mux2/6  "Mot_RR"
  Read CM Dict9/1 -> Mux2/7
  Read CM Dict3/1 -> Radians to Degrees/1
  Read CM Dict4/1 -> Radians to Degrees1/1
  Radians to Degrees/1 -> Add/1
  Radians to Degrees1/1 -> Add/2
  Radians to Degrees2/1 -> Data Type Conversion5/1, Mux4/1, Mux2/2  "r"
  Radians to Degrees3/1 -> Mux2/1  "r_ref"
  Add/1 -> Gain/1
  Mux2/1 -> To File/1
  Read CM Dict1/1 -> Mux2/9
  Read CM Dict5/1 -> Mux2/10
  Rate Transition/1 -> Data Type Conversion/1
  Mux4/1 -> "crossplotrsteer "/1
  Gain/1 -> Mux2/8, Mux4/2  "steering"
  Bus Selector4/1 -> Rate Transition1/1  "<FL>"
  Bus Selector4/2 -> Rate Transition2/1  "<FR>"
  Bus Selector4/3 -> Rate Transition3/1  "<RL>"
  Bus Selector4/4 -> Rate Transition4/1  "<RR>"
  SR/1 -> Bus Selector4/1
  Rate Transition1/1 -> Data Type Conversion1/1
  Rate Transition2/1 -> Data Type Conversion2/1
  Rate Transition3/1 -> Data Type Conversion3/1
  Rate Transition4/1 -> Data Type Conversion4/1
  Data Type Conversion1/1 -> Mux2/11
  Data Type Conversion2/1 -> Mux2/12
  Data Type Conversion3/1 -> Mux2/13
  Data Type Conversion4/1 -> Mux2/14
  Gain7/1 -> Gain9/1
  Gain9/1 -> Mux2/15  "Motor_RPM"
  Read CM Dict24/1 -> Gain7/1
  Read CM Dict25/1 -> Gain10/1
  Gain10/1 -> Gain11/1
  Gain11/1 -> Mux2/16  "Motor_RPM"
  Gain12/1 -> Gain13/1
  Gain13/1 -> Mux2/17  "Motor_RPM"
  Gain14/1 -> Gain15/1
  Gain15/1 -> Mux2/18  "Motor_RPM"
  Read CM Dict26/1 -> Gain12/1
  Read CM Dict27/1 -> Gain14/1
  Read CM Dict10/1 -> Gain1/1
  Gain1/1 -> Mux2/19
  Read CM Dict20/1 -> Radians to Degrees4/1
  Data Type Conversion47/1 -> Mux1/1  "steer"
  Mux1/1 -> crossplotrsteer 1/1
  Radians to Degrees4/1 -> Data Type Conversion47/1
  Data Type Conversion5/1 -> Mux1/2  "r"
  Read CM Dict6/1 -> Radians to Degrees5/1
  Radians to Degrees5/1 -> Mux2/20
